simulink model "test"  (Simulink 7.9)
settings: Solver=ode45  StartTime=0.0  StopTime=10.0  RelTol=1e-3
values from neighbouring files (symbols this model uses):
  magic = 0.0004748    [cmodel_data.m]
  radius = 0.579106    [2xPol.m]    (also in cmodel_data.m = 0.6)
  T = 0.01695    [cmodel_data.m]
settings Model: Creator=ex16  LastModifiedBy=ex16

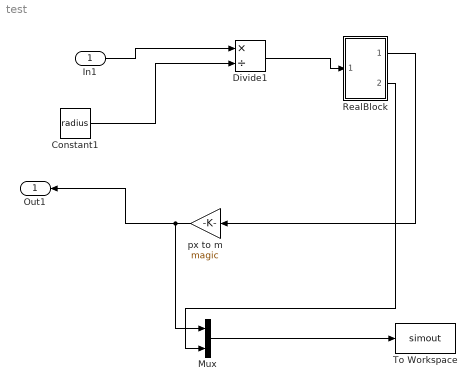
== system test ==
  In1 : Inport  SampleTime=T
  Constant1 : Constant  Value=radius
  Divide1 : Product  Inputs=*/
  Mux : Mux  Inputs=2
  RealBlock : Subsystem
  To Workspace : ToWorkspace  VariableName=simout  SampleTime=-1  SaveFormat=Structure With Time
  px to m : Gain  Gain=magic
  Out1 : Outport
  wires:
  Constant1/1 -> Divide1/2
  In1/1 -> Divide1/1
  px to m/1 -> Out1/1, Mux/1
  RealBlock/1(Out1) -> px to m/1
  Divide1/1 -> RealBlock/1(In1)
  Mux/1 -> To Workspace/1
  RealBlock/2(Scope) -> Mux/2

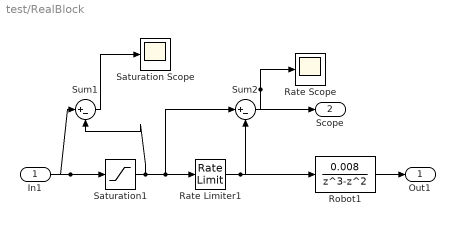
== system test/RealBlock ==
  In1 : Inport
  Rate Limiter1 : RateLimiter  RisingSlewLimit=15  FallingSlewLimit=-15  SampleTimeMode=inherited
  Rate Scope : Scope
      settings: TimeRange=2  YMin=0  YMax=0.25  SaveName=ScopeData2
  Robot1 : DiscreteTransferFcn  Numerator=[0.008]  Denominator=[1 -1 0 0]  SampleTime=T
  Saturation Scope : Scope
  Saturation1 : Saturate  UpperLimit=3.2  LowerLimit=-3.2  SampleTime=T
  Sum1 : Sum  Inputs=|+-
  Sum2 : Sum  Inputs=|+-
  Out1 : Outport
  Scope : Outport  Port=2
  wires:
  Saturation1/1 -> Rate Limiter1/1, Sum2/1, Sum1/2
  Rate Limiter1/1 -> Robot1/1, Sum2/2
  Sum2/1 -> Rate Scope/1, Scope/1
  Robot1/1 -> Out1/1
  In1/1 -> Saturation1/1, Sum1/1
  Sum1/1 -> Saturation Scope/1
